simulink model "practica3"  (R2015a)
settings: Solver=ode4  StartTime=0.0  StopTime=5  FixedStep=.01  RelTol=1e-3
settings Model: Creator=Sala6  LastModifiedBy=Sala6

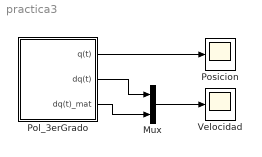
== system practica3 ==
  Mux : Mux  Inputs=2
  Pol_3erGrado : Subsystem  mask{t0=0, tf=5, q0=4, qf=20, v0=-5, vf=10}
      mask prompts: t0 "Tiempo inicial"; tf "Tiempo final"; q0 "Posicion inicial"; qf "Posicion final"; v0 "Velocidad inicial"; vf "Velocidad final"
      mask init:
      | A=[1 t0 t0^2 t0^3;0 1 2*t0 3*t0^2;1 tf tf^2 tf^3;0 1 2*tf 3*tf^2];
      | b=[q0;v0;qf;vf];
      | x=inv(A)*b;
      | a0=x(1);
      | a1=x(2);
      | a2=x(3);
      | a3=x(4);
  Posicion : Scope
  Velocidad : Scope
  wires:
  Mux/1 -> Velocidad/1
  Pol_3erGrado/1(q(t)) -> Posicion/1
  Pol_3erGrado/2(dq(t)) -> Mux/1
  Pol_3erGrado/3(dq(t)_mat) -> Mux/2

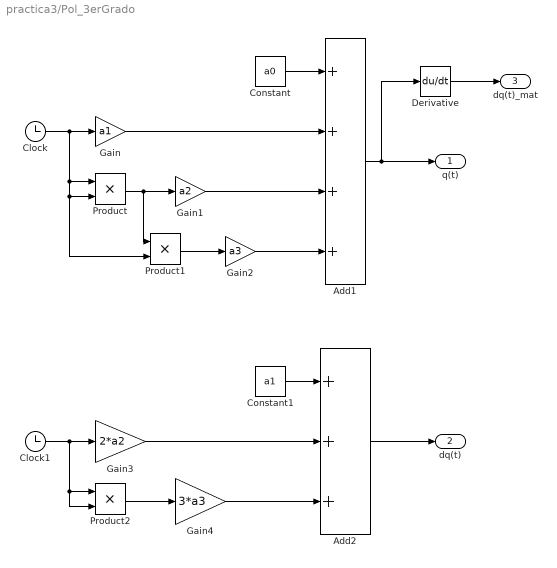
== system practica3/Pol_3erGrado ==
  Add1 : Sum  Inputs=++++
  Add2 : Sum  Inputs=+++
  Clock : Clock
  Clock1 : Clock
  Constant : Constant  Value=a0
  Constant1 : Constant  Value=a1
  Derivative : Derivative
  Gain : Gain  Gain=a1
  Gain1 : Gain  Gain=a2
  Gain2 : Gain  Gain=a3
  Gain3 : Gain  Gain=2*a2
  Gain4 : Gain  Gain=3*a3
  Product : Product
  Product1 : Product
  Product2 : Product
  q(t) : Outport
  dq(t) : Outport  Port=2
  dq(t)_mat : Outport  Port=3
  wires:
  Clock/1 -> Product1/2, Product/2, Product/1, Gain/1
  Gain3/1 -> Add2/2
  Gain2/1 -> Add1/4
  Constant/1 -> Add1/1
  Gain/1 -> Add1/2
  Product2/1 -> Gain4/1
  Product/1 -> Product1/1, Gain1/1
  Clock1/1 -> Gain3/1, Product2/1, Product2/2
  Product1/1 -> Gain2/1
  Gain4/1 -> Add2/3
  Add1/1 -> q(t)/1, Derivative/1
  Constant1/1 -> Add2/1
  Add2/1 -> dq(t)/1
  Gain1/1 -> Add1/3
  Derivative/1 -> dq(t)_mat/1
